simulink model "Simulink_Fuzzy"  (Simulink 8.3)
settings: Solver=ode3  StartTime=0.0  StopTime=10.0  RelTol=1e-3
libraries: fuzblock x1, simulink x1
settings Model: Creator=Usuario  LastModifiedBy=Lab Man
settings OptimizationCC: ExpressionDepthLimit=2147483647
settings DebuggingCC: FcnCallInpInsideContextMsg=UseLocalSettings

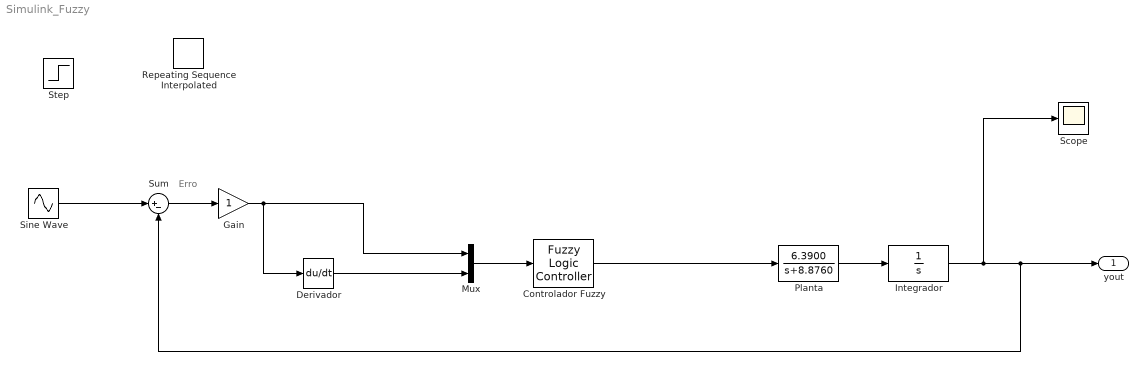
== system Simulink_Fuzzy ==
  note: Erro
  Controlador Fuzzy : fuzblock/Fuzzy Logic  Controller  fis=FuzzyFinal
  Derivador : Derivative
  Gain : Gain
  Integrador : TransferFcn  Denominator=[1 0]
  Mux : Mux  Inputs=2
  Planta : TransferFcn  Numerator=[6.3900]  Denominator=[1 8.8760]
  Repeating Sequence Interpolated : simulink/Sources/Repeating Sequence Interpolated  OutValues=[0 0.1 0.2 0.2 0.2 0.2 0.2 0.5 0.5] .'  TimeValues=[0 1 2 3 4 5 6 6.1 10].'  LookUpMeth=Interpolation-Use End Values  tsamp=0.01  OutMin=[]  OutMax=[]  OutDataTypeStr=double  OutputDataTypeScalingMode=double  OutDataType=fixdt(0,8)  OutScaling=2^-10
  Scope : Scope
  Sine Wave : Sin  SampleTime=0
  Step : Step  Time=0  SampleTime=0.05
  Sum : Sum  Inputs=|+-
  yout : Outport
  wires:
  Planta/1 -> Integrador/1
  Gain/1 -> Mux/1, Derivador/1
  Sum/1 -> Gain/1
  Mux/1 -> Controlador Fuzzy/1
  Derivador/1 -> Mux/2
  Integrador/1 -> Scope/1, yout/1, Sum/2
  Controlador Fuzzy/1 -> Planta/1
  Sine Wave/1 -> Sum/1
